simulink model "ApproximateAdder"  (R2020b)
settings: Solver=VariableStepAuto  StartTime=0.0  StopTime=1024  RelTol=1e-3
libraries: xbsIndex_r4 x195
settings Model: Creator=666sk  LastModifiedBy=666sk

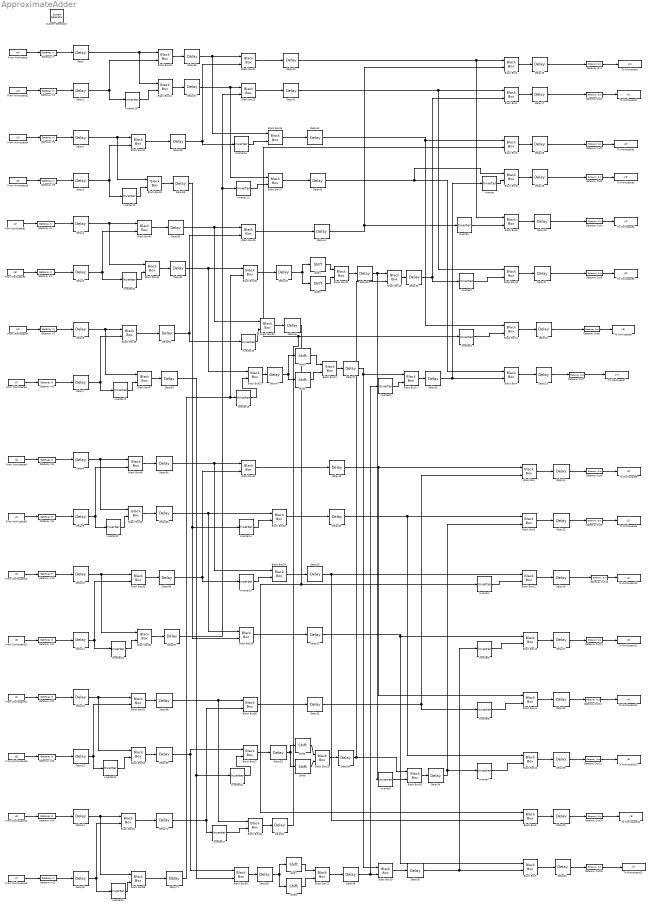
== system ApproximateAdder ==
  " System Generator" : xbsIndex_r4/ System Generator  Tag=genX  xilinxfamily=artix7  part=xc7a100t  speed=-1  package=csg324  synthesis_tool=Vivado  clock_wrapper=Clock Enables  directory=C:/Users/666sk/Desktop  proj_type=Vivado  Synth_file=Vivado Synthesis Defaults  Impl_file=Vivado Implementation Defaults  testbench=off  simulink_period=1  sysclk_period=5  dcm_input_clock_period=10  incr_netlist=off  trim_vbits=Everywhere in SubSystem  dbl_ovrd=According to Block Masks  core_generation=According to Block Masks  run_coregen=off  deprecated_control=off  eval_field=0  block_type=sysgen
  Black Box{,1..55} (56 alike) : xbsIndex_r4/Black Box  init_code=adder_8_bits_config  sim_method=ISE Simulator  verbose=off  block_type=blackbox2
  Delay{,1..15,32..39,45,47,53,55..71} (44 alike) : xbsIndex_r4/Delay  rst=off  infoeditControl=Selection of Reset will increase slice count due to use of real FFs and instead of SRLs  en=off  latency=1  reg_retiming=off  dbl_ovrd=off  block_type=delay
  Delay{16..31} (16 alike) : xbsIndex_r4/Delay  rst=off  infoeditControl=Selection of Reset will increase slice count due to use of real FFs and instead of SRLs  en=off  latency=2  reg_retiming=off  dbl_ovrd=off  block_type=delay
  Delay{40..44,46,48..52,54} (12 alike) : xbsIndex_r4/Delay  rst=off  infoeditControl=Selection of Reset will increase slice count due to use of real FFs and instead of SRLs  en=off  latency=3  reg_retiming=off  dbl_ovrd=off  block_type=delay
  From Workspace : FromWorkspace  VariableName=v0r
  From Workspace1 : FromWorkspace  VariableName=v1r
  From Workspace10 : FromWorkspace  VariableName=v2i
  From Workspace11 : FromWorkspace  VariableName=v6i
  From Workspace12 : FromWorkspace  VariableName=v1i
  From Workspace13 : FromWorkspace  VariableName=v5i
  From Workspace14 : FromWorkspace  VariableName=v3i
  From Workspace15 : FromWorkspace  VariableName=v7i
  From Workspace2 : FromWorkspace  VariableName=v4r
  From Workspace3 : FromWorkspace  VariableName=v5r
  From Workspace4 : FromWorkspace  VariableName=v2r
  From Workspace5 : FromWorkspace  VariableName=v7r
  From Workspace6 : FromWorkspace  VariableName=v6r
  From Workspace7 : FromWorkspace  VariableName=v3r
  From Workspace8 : FromWorkspace  VariableName=v0i
  From Workspace9 : FromWorkspace  VariableName=v4i
  Gateway In{,1..15} (16 alike) : xbsIndex_r4/Gateway In  gui_display_data_type=Fixed-point  arith_type="Signed  (2's comp)"  n_bits=WIN  bin_pt=DIN  preci_type=Single  exp_width=8  frac_width=24  rows=1  columns=1  quantization="Round  (unbiased: +/- Inf)"  overflow=Saturate  period=1  UseAsADC=off  ADCChannel='1'  interface=None  automatic_assignment=on  address_offset=hex2dec('00')  intf_name=''  intf_description=''  default_value=0  timing_constraint=None  locs_specified=off  LOCs={}  io_standard={}  inherit_from_input=off  hdl_port=on  dbl_ovrd=off  block_type=gatewayin
  Gateway Out{,1..15} (16 alike) : xbsIndex_r4/Gateway Out  inherit_from_input=off  hdl_port=on  rows=1  columns=1  UseAsDAC=off  DACChannel='1'  interface=None  automatic_assignment=on  address_offset=hex2dec('00')  intf_name=''  intf_description=''  timing_constraint=None  locs_specified=off  LOCs={}  io_standard={}  block_type=gatewayout
  Inverter{,1..25} (26 alike) : xbsIndex_r4/Inverter  en=off  latency=0  dbl_ovrd=off  block_type=inv
  Shift{1,3,5,7} (4 alike) : xbsIndex_r4/Shift  shift_dir=Right  shift_bits=1  en=off  latency=0  precision=Full  arith_type="Signed  (2's comp)"  n_bits=16  bin_pt=14  quantization=Truncate  overflow=Wrap  dbl_ovrd=off  block_type=shift
  Shift{2,4,6,8} (4 alike) : xbsIndex_r4/Shift  shift_dir=Right  shift_bits=2  en=off  latency=0  precision=Full  arith_type="Signed  (2's comp)"  n_bits=16  bin_pt=14  quantization=Truncate  overflow=Wrap  dbl_ovrd=off  block_type=shift
  To Workspace : ToWorkspace  VariableName=y0r  SaveFormat=Timeseries  SampleTime=-1
  To Workspace1 : ToWorkspace  VariableName=y1r  SaveFormat=Timeseries  SampleTime=-1
  To Workspace10 : ToWorkspace  VariableName=y2i  SaveFormat=Timeseries  SampleTime=-1
  To Workspace11 : ToWorkspace  VariableName=y3i  SaveFormat=Timeseries  SampleTime=-1
  To Workspace12 : ToWorkspace  VariableName=y4i  SaveFormat=Timeseries  SampleTime=-1
  To Workspace13 : ToWorkspace  VariableName=y5i  SaveFormat=Timeseries  SampleTime=-1
  To Workspace14 : ToWorkspace  VariableName=y6i  SaveFormat=Timeseries  SampleTime=-1
  To Workspace15 : ToWorkspace  VariableName=y7i  SaveFormat=Timeseries  SampleTime=-1
  To Workspace2 : ToWorkspace  VariableName=y2r  SaveFormat=Timeseries  SampleTime=-1
  To Workspace3 : ToWorkspace  VariableName=y3r  SaveFormat=Timeseries  SampleTime=-1
  To Workspace4 : ToWorkspace  VariableName=y4r  SaveFormat=Timeseries  SampleTime=-1
  To Workspace5 : ToWorkspace  VariableName=y5r  SaveFormat=Timeseries  SampleTime=-1
  To Workspace6 : ToWorkspace  VariableName=y6r  SaveFormat=Timeseries  SampleTime=-1
  To Workspace7 : ToWorkspace  VariableName=y7r  SaveFormat=Timeseries  SampleTime=-1
  To Workspace8 : ToWorkspace  VariableName=y0i  SaveFormat=Timeseries  SampleTime=-1
  To Workspace9 : ToWorkspace  VariableName=y1i  SaveFormat=Timeseries  SampleTime=-1
  wires:
  Black Box40/1 -> Delay56/1
  Delay31/1 -> Gateway Out15/1
  Gateway In13/1 -> Delay13/1
  Delay25/1 -> Gateway Out9/1
  From Workspace13/1 -> Gateway In13/1
  Shift8/1 -> Black Box22/2
  Shift5/1 -> Black Box23/1
  Delay26/1 -> Gateway Out10/1
  From Workspace4/1 -> Gateway In4/1
  Gateway In2/1 -> Delay1/1
  Delay6/1 -> Black Box47/1, Black Box46/1
  Delay1/1 -> Inverter18/1, Black Box40/2
  Gateway Out8/1 -> To Workspace8/1
  Black Box11/1 -> Delay22/1
  From Workspace8/1 -> Gateway In8/1
  Black Box8/1 -> Delay19/1
  Gateway Out6/1 -> To Workspace6/1
  From Workspace/1 -> Gateway In/1
  Delay18/1 -> Gateway Out2/1
  Delay21/1 -> Gateway Out5/1
  Delay67/1 -> Black Box25/2, Inverter11/1
  Black Box32/1 -> Delay48/1
  From Workspace10/1 -> Gateway In10/1
  Black Box12/1 -> Delay26/1
  Black Box16/1 -> Delay32/1
  Gateway In10/1 -> Delay10/1
  Delay4/1 -> Black Box45/1, Black Box44/1
  Gateway Out7/1 -> To Workspace7/1
  Delay3/1 -> Inverter19/1, Black Box42/2
  Gateway Out5/1 -> To Workspace5/1
  Delay63/1 -> Black Box39/2, Inverter16/1
  Delay10/1 -> Black Box51/1, Black Box50/1
  Gateway In7/1 -> Delay6/1
  Delay46/1 -> Black Box6/1, Inverter4/1
  Delay27/1 -> Gateway Out11/1
  Black Box36/1 -> Delay52/1
  Gateway Out11/1 -> To Workspace11/1
  Black Box43/1 -> Delay59/1
  Black Box45/1 -> Delay61/1
  Black Box28/1 -> Delay44/1
  Delay19/1 -> Gateway Out3/1
  Gateway In4/1 -> Delay2/1
  Shift3/1 -> Black Box21/1
  Gateway In6/1 -> Delay3/1
  Gateway Out12/1 -> To Workspace12/1
  Black Box2/1 -> Delay17/1
  Gateway In1/1 -> Delay4/1
  Gateway In5/1 -> Delay7/1
  Delay33/1 -> Inverter/1, Black Box4/2
  Shift1/1 -> Black Box20/1
  Gateway Out13/1 -> To Workspace13/1
  Black Box35/1 -> Delay51/1
  Delay68/1 -> Black Box38/1, Black Box36/1
  Gateway Out2/1 -> To Workspace2/1
  Black Box55/1 -> Delay71/1
  Shift6/1 -> Black Box23/2
  Delay8/1 -> Black Box49/1, Black Box48/1
  From Workspace6/1 -> Gateway In6/1
  Delay5/1 -> Inverter20/1, Black Box44/2
  Black Box42/1 -> Delay58/1
  Delay2/1 -> Black Box43/1, Black Box42/1
  Delay11/1 -> Inverter23/1, Black Box50/2
  Shift7/1 -> Black Box22/1
  Delay65/1 -> Black Box35/1, Black Box33/1
  Delay30/1 -> Gateway Out14/1
  Delay29/1 -> Gateway Out13/1
  Delay64/1 -> Black Box34/1, Black Box32/1
  From Workspace2/1 -> Gateway In2/1
  Gateway In3/1 -> Delay5/1
  From Workspace1/1 -> Gateway In1/1
  Black Box/1 -> Delay24/1
  Delay70/1 -> Inverter17/1, Black Box36/2
  Delay20/1 -> Gateway Out4/1
  Black Box5/1 -> Delay25/1
  Black Box25/1 -> Delay41/1
  Shift2/1 -> Black Box20/2
  Delay7/1 -> Inverter21/1, Black Box46/2
  Gateway In8/1 -> Delay8/1
  Delay16/1 -> Gateway Out/1
  Delay23/1 -> Gateway Out7/1
  Gateway In12/1 -> Delay12/1
  Gateway In9/1 -> Delay9/1
  Delay14/1 -> Black Box55/1, Black Box54/1
  Delay24/1 -> Gateway Out8/1
  Black Box41/1 -> Delay57/1
  Black Box34/1 -> Delay50/1
  Delay69/1 -> Black Box37/1, Black Box39/1
  Delay38/1 -> Black Box18/1, Black Box16/2
  Delay/1 -> Black Box41/1, Black Box40/1
  Black Box19/1 -> Delay35/1
  Black Box33/1 -> Delay49/1
  Black Box4/1 -> Delay23/1
  Black Box44/1 -> Delay60/1
  From Workspace9/1 -> Gateway In9/1
  Black Box20/1 -> Delay36/1
  From Workspace3/1 -> Gateway In3/1
  Gateway Out1/1 -> To Workspace1/1
  Delay9/1 -> Inverter22/1, Black Box48/2
  From Workspace14/1 -> Gateway In14/1
  Gateway In/1 -> Delay/1
  Black Box1/1 -> Delay16/1
  Black Box22/1 -> Delay39/1
  From Workspace5/1 -> Gateway In5/1
  Black Box38/1 -> Delay54/1
  Gateway In14/1 -> Delay14/1
  Delay66/1 -> Inverter15/1, Black Box32/2
  Delay17/1 -> Gateway Out1/1
  Black Box24/1 -> Delay40/1
  Delay15/1 -> Inverter25/1, Black Box54/2
  Black Box26/1 -> Delay42/1
  Gateway Out9/1 -> To Workspace9/1
  Delay22/1 -> Gateway Out6/1
  Black Box27/1 -> Delay43/1
  Black Box6/1 -> Delay30/1
  Gateway Out4/1 -> To Workspace4/1
  Black Box13/1 -> Delay27/1
  Gateway In15/1 -> Delay15/1
  From Workspace12/1 -> Gateway In12/1
  Gateway Out/1 -> To Workspace/1
  Gateway Out14/1 -> To Workspace14/1
  Gateway Out3/1 -> To Workspace3/1
  Delay28/1 -> Gateway Out12/1
  Delay12/1 -> Black Box53/1, Black Box52/1
  Black Box15/1 -> Delay29/1
  Gateway In11/1 -> Delay11/1
  Black Box21/1 -> Delay37/1
  Black Box9/1 -> Delay20/1
  Black Box7/1 -> Delay31/1
  Shift4/1 -> Black Box21/2
  From Workspace11/1 -> Gateway In11/1
  From Workspace15/1 -> Gateway In15/1
  From Workspace7/1 -> Gateway In7/1
  Delay13/1 -> Inverter24/1, Black Box52/2
  Black Box3/1 -> Delay18/1
  Delay34/1 -> Black Box5/2, Inverter7/1
  Black Box14/1 -> Delay28/1
  Gateway Out10/1 -> To Workspace10/1
  Black Box10/1 -> Delay21/1
  Gateway Out15/1 -> To Workspace15/1
  Inverter/1 -> Black Box8/2
  Inverter1/1 -> Black Box9/2
  Inverter2/1 -> Black Box10/2
  Inverter3/1 -> Black Box11/2
  Inverter4/1 -> Black Box12/2
  Inverter5/1 -> Black Box13/2
  Inverter6/1 -> Black Box14/2
  Inverter7/1 -> Black Box15/2
  Delay32/1 -> Inverter2/1, Black Box2/2
  Inverter8/1 -> Black Box17/2
  Black Box17/1 -> Delay33/1
  Inverter9/1 -> Black Box18/2
  Black Box18/1 -> Delay34/1
  Delay35/1 -> Inverter5/1, Black Box7/2
  Delay36/1 -> Black Box16/1, Inverter9/1
  Delay37/1 -> Black Box19/1, Black Box17/1
  Delay39/1 -> Black Box19/2, Inverter8/1
  Black Box23/1 -> Delay38/1
  Delay40/1 -> Black Box9/1, Black Box1/1
  Delay41/1 -> Black Box10/1, Black Box2/1
  Delay42/1 -> Black Box11/1, Black Box3/1
  Inverter10/1 -> Black Box26/2
  Delay43/1 -> Black Box8/1, Black Box4/1
  Inverter11/1 -> Black Box27/2
  Delay44/1 -> Inverter1/1, Black Box1/2
  Delay45/1 -> Shift2/1, Shift1/1
  Black Box29/1 -> Delay45/1
  Black Box30/1 -> Delay46/1
  Inverter12/1 -> Black Box30/2
  Inverter13/1 -> Black Box31/2
  Black Box31/1 -> Delay47/1
  Delay47/1 -> Shift3/1, Shift4/1
  Delay48/1 -> Black Box14/1, Black Box/1
  Delay49/1 -> Black Box15/1, Black Box5/1
  Inverter14/1 -> Black Box33/2
  Delay50/1 -> Black Box12/1, Black Box6/2
  Inverter15/1 -> Black Box34/2
  Delay51/1 -> Black Box13/1, Black Box7/1
  Delay52/1 -> Inverter6/1, Black Box/2
  Delay53/1 -> Shift6/1, Shift5/1
  Black Box37/1 -> Delay53/1
  Inverter16/1 -> Black Box37/2
  Delay54/1 -> Black Box3/2, Inverter3/1
  Inverter17/1 -> Black Box38/2
  Black Box39/1 -> Delay55/1
  Delay55/1 -> Shift8/1, Shift7/1
  Delay56/1 -> Black Box26/1, Black Box24/1
  Delay57/1 -> Black Box27/1, Black Box25/1
  Inverter18/1 -> Black Box41/2
  Delay58/1 -> Inverter10/1, Black Box24/2
  Delay59/1 -> Black Box35/2, Inverter14/1
  Inverter19/1 -> Black Box43/2
  Delay61/1 -> Black Box31/1, Black Box29/1
  Delay60/1 -> Black Box30/1, Black Box28/1
  Inverter20/1 -> Black Box45/2
  Delay62/1 -> Black Box28/2, Inverter12/1
  Black Box46/1 -> Delay62/1
  Black Box47/1 -> Delay63/1
  Inverter21/1 -> Black Box47/2
  Black Box48/1 -> Delay64/1
  Black Box49/1 -> Delay65/1
  Inverter22/1 -> Black Box49/2
  Black Box50/1 -> Delay66/1
  Black Box51/1 -> Delay67/1
  Inverter23/1 -> Black Box51/2
  Black Box52/1 -> Delay68/1
  Inverter24/1 -> Black Box53/2
  Black Box53/1 -> Delay69/1
  Black Box54/1 -> Delay70/1
  Delay71/1 -> Black Box29/2, Inverter13/1
  Inverter25/1 -> Black Box55/2
